simulink library "lib_Gimbal_Ctrl"  (R2017a)
settings: Solver=VariableStepAuto  StartTime=0.0  StopTime=10.0  RelTol=1e-3
undefined symbols (not defined in the file or in its folder): FT_HWI_CC_Data, Standard_Devices, UDP_Protocol
undefined symbols (not defined in the file): HIL_Data
libraries: simulink x19, sldrtlib x2
(part 1 of 2)
settings Model: Creator=m.hiepp  LastModifiedBy=m.hiepp
settings SFSimCC: SimUseLocalCustomCode=on
settings RTWCC: RTWUseLocalCustomCode=on

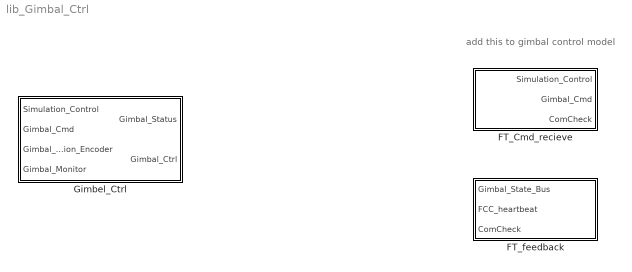
== system lib_Gimbal_Ctrl ==
  note: add this to gimbal control model
  FT_Cmd_recieve : Subsystem
  FT_feedback : Subsystem
  Gimbel_Ctrl : Subsystem  mask{Gimbal_Ctrl=HIL_Data.Gimbal_Ctrl, SampTime=HIL_Data.Gimbal_Ctrl.SampTime}
      mask prompts: SampTime "Sample Time"

== system lib_Gimbal_Ctrl/FT_Cmd_recieve ==
  note: serves also as hold when there is no new input!
  Construct_Busses : Subsystem
  Logical Operator : Logic  AllPortsSameDT=off  OutDataTypeStr=boolean
  NOT : Logic  Operator=NOT  IconShape=distinctive  AllPortsSameDT=off  OutDataTypeStr=boolean
  Receive_from_SimulationPC : sldrtlib/Packet Input  SampleTime=FT_HWI_CC_Data.SampTime  MaxMissedTicks=FT_HWI_CC_Data.MaxMissTicks  ShowMissedTicks=off  YieldWhenWaiting=on  DrvName=Standard_Devices/UDP_Protocol  DrvAddress=36880  DrvOptions=[3232235970 36864]  PacketSize=52  DataTypes={'boolean','boolean','double','double','uint16','double','double','double','double'}  ShowReady=on  ShowError=on  PacketID=1  ByteOrder=1  ShowTimestamp=off
      settings: AttributesFormatString=UDP Protocol [36880]  SourceProductName=Simulink Desktop Real-Time
  Simulation_Control : Outport  OutDataTypeStr=Bus: Simulation_Ctrl_Bus
  Gimbal_Cmd : Outport  Port=2  OutDataTypeStr=Bus: Gimbal_Cmd_Bus
  ComCheck : Outport  Port=3
  wires:
  Receive_from_SimulationPC/8 -> Construct_Busses/8(GimCmd_psi)  "Gimbal_Psi_Cmd_deg"
  Receive_from_SimulationPC/7 -> Construct_Busses/7(GimCmd_theta)  "Gimbal_Theta_Cmd_deg"
  Receive_from_SimulationPC/6 -> Construct_Busses/6(GimCmd_phi)  "Gimbal_Phi_Cmd_deg"
  Receive_from_SimulationPC/4 -> Construct_Busses/4(SimCtrl_gimbal_flg)  "stop_gimbal_flg"
  Receive_from_SimulationPC/3 -> Construct_Busses/3(SimCtrl_enable_gimbal_flg)  "enable_gimbal_ctrl_flg"
  Receive_from_SimulationPC/2 -> Construct_Busses/2(SimCtrl_reset)  "reset"
  Receive_from_SimulationPC/1 -> Construct_Busses/1(SimCtrl_run)  "run"
  Construct_Busses/2(Gimbal_Cmd) -> Gimbal_Cmd/1
  Construct_Busses/1(Simulation_Control) -> Simulation_Control/1
  Receive_from_SimulationPC/5 -> Construct_Busses/5(SimCtrl_heartbeat)  "Gimbal_Phi_Cmd_deg"
  NOT/1 -> Logical Operator/2
  Logical Operator/1 -> Construct_Busses/Enable
  Receive_from_SimulationPC/10 -> Logical Operator/1  "DataReady_flg"
  Receive_from_SimulationPC/11 -> NOT/1  "DataError_flg"
  Receive_from_SimulationPC/9 -> Construct_Busses/9(ComCheck_update)  "ComCheck"
  Construct_Busses/3(ComCheck) -> ComCheck/1

== system lib_Gimbal_Ctrl/FT_feedback ==
  note: only relevant signals are transfered
  Gimbal_State_Bus : Inport  OutDataTypeStr=Bus: Gimbal_State_Bus
  FCC_heartbeat : Inport  Port=2
  ComCheck : Inport  Port=3
  Bus Selector : BusSelector  OutputSignals=Gimbal_Status.Gimbal_operational_flg,Gimbal_Status.Gimbal_Ramp_flg,Gimbal_Status.Gimbal_Limit_flg,Gimbal_Status.Gimbal_StopSim_flg,Gimbal_Encoder_Signals.ATT_Gimbal.Gimbal_yaw_sns,Gimbal_Encoder_Signals.ATT_Gimbal.Gimbal_pitch_sns,Gimbal_Encoder_Signals.ATT_Gimbal.Gimbal_roll_sns
  Compare To Constant : simulink/Logic and Bit Operations/Compare To Constant  relop===  const=FT_HWI_CC_Data.ComFreq_mark  OutDataTypeStr=boolean
  Counter Limited : simulink/Sources/Counter Limited  uplimit=FT_HWI_CC_Data.ComFreq_mark  tsamp=FT_HWI_CC_Data.SampTime
  send_FB : Subsystem
  wires:
  Gimbal_State_Bus/1 -> Bus Selector/1
  Counter Limited/1 -> Compare To Constant/1
  Bus Selector/1 -> send_FB/1(Gimbal_operational_flg)  "<Gimbal_operational_flg>"
  Bus Selector/2 -> send_FB/2(Gimbal_Ramp_flg)  "<Gimbal_Ramp_flg>"
  Bus Selector/3 -> send_FB/3(Gimbal_Limit_flg)  "<Gimbal_Limit_flg>"
  Bus Selector/4 -> send_FB/4(Gimbal_StopSim_flg)  "<Gimbal_StopSim_flg>"
  Bus Selector/5 -> send_FB/5(Gimbal_yaw_sns)  "<Gimbal_yaw_sns>"
  Bus Selector/6 -> send_FB/6(Gimbal_pitch_sns)  "<Gimbal_pitch_sns>"
  Bus Selector/7 -> send_FB/7(Gimbal_roll_sns)  "<Gimbal_roll_sns>"
  Compare To Constant/1 -> send_FB/Enable
  FCC_heartbeat/1 -> send_FB/8(FCC_heartbeat)
  ComCheck/1 -> send_FB/9(ComCheck)

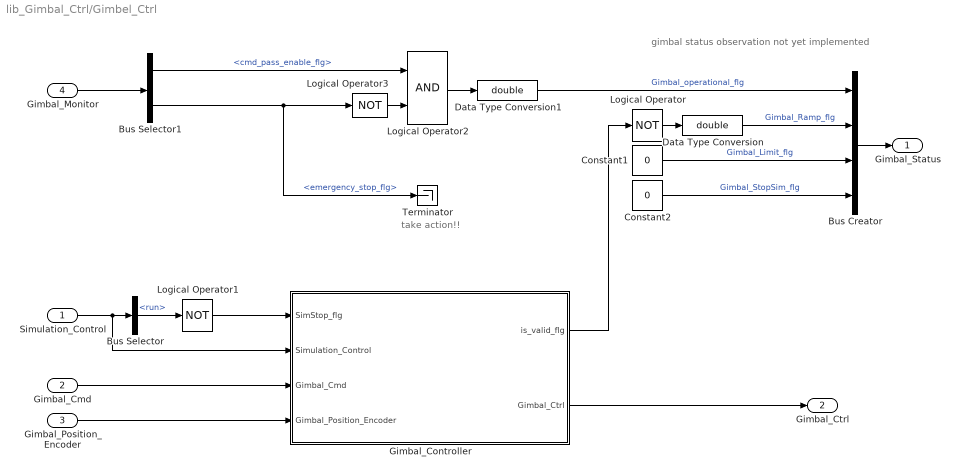
== system lib_Gimbal_Ctrl/Gimbel_Ctrl ==
  note: take action!!
  note: gimbal status observation not yet implemented
  Simulation_Control : Inport  OutDataTypeStr=Bus: Simulation_Ctrl_Bus
  Gimbal_Cmd : Inport  Port=2  OutDataTypeStr=Bus: Gimbal_Cmd_Bus
  Gimbal_Position_Encoder : Inport  Port=3  OutDataTypeStr=Bus: Gimbal_Encoder_Bus
  Gimbal_Monitor : Inport  Port=4  OutDataTypeStr=Bus: Gimbal_Monitor_Bus
  Bus Creator : BusCreator  Inputs=4
  Bus Selector : BusSelector  OutputSignals=run
  Bus Selector1 : BusSelector  OutputSignals=cmd_pass_enable_flg,emergency_stop_flg
  Constant1 : Constant  Value=0
  Constant2 : Constant  Value=0
  Data Type Conversion : DataTypeConversion  OutDataTypeStr=double
  Data Type Conversion1 : DataTypeConversion  OutDataTypeStr=double
  Gimbal_Controller : Subsystem
  Logical Operator : Logic  Operator=NOT  AllPortsSameDT=off  OutDataTypeStr=boolean
  Logical Operator1 : Logic  Operator=NOT  AllPortsSameDT=off  OutDataTypeStr=boolean
  Logical Operator2 : Logic  AllPortsSameDT=off  OutDataTypeStr=boolean
  Logical Operator3 : Logic  Operator=NOT  AllPortsSameDT=off  OutDataTypeStr=boolean
  Terminator : Terminator
  Gimbal_Status : Outport  OutDataTypeStr=Bus: Gimbal_Status_Bus
  Gimbal_Ctrl : Outport  Port=2  OutDataTypeStr=Bus: Gimbal_Ctrl_Bus
  wires:
  Bus Creator/1 -> Gimbal_Status/1
  Logical Operator/1 -> Data Type Conversion/1
  Gimbal_Controller/2(Gimbal_Ctrl) -> Gimbal_Ctrl/1
  Gimbal_Controller/1(is_valid_flg) -> Logical Operator/1
  Simulation_Control/1 -> Gimbal_Controller/2(Simulation_Control), Bus Selector/1
  Gimbal_Position_Encoder/1 -> Gimbal_Controller/4(Gimbal_Position_Encoder)
  Gimbal_Cmd/1 -> Gimbal_Controller/3(Gimbal_Cmd)
  Bus Selector/1 -> Logical Operator1/1  "<run>"
  Logical Operator1/1 -> Gimbal_Controller/1(SimStop_flg)
  Data Type Conversion1/1 -> Bus Creator/1  "Gimbal_operational_flg"
  Constant1/1 -> Bus Creator/3  "Gimbal_Limit_flg"
  Constant2/1 -> Bus Creator/4  "Gimbal_StopSim_flg"
  Data Type Conversion/1 -> Bus Creator/2  "Gimbal_Ramp_flg"
  Gimbal_Monitor/1 -> Bus Selector1/1
  Bus Selector1/1 -> Logical Operator2/1  "<cmd_pass_enable_flg>"
  Bus Selector1/2 -> Terminator/1, Logical Operator3/1  "<emergency_stop_flg>"
  Logical Operator2/1 -> Data Type Conversion1/1
  Logical Operator3/1 -> Logical Operator2/2

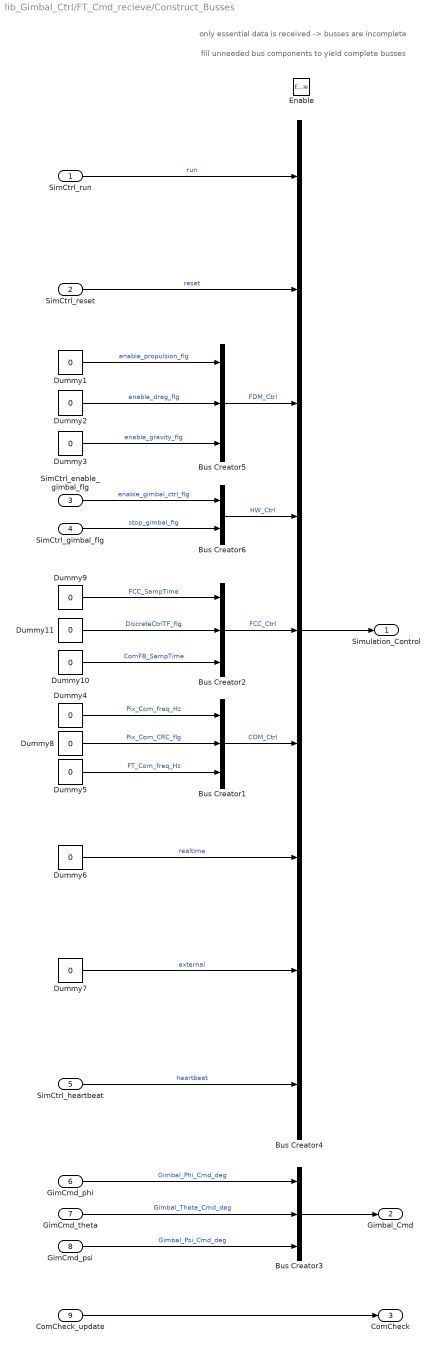
== system lib_Gimbal_Ctrl/FT_Cmd_recieve/Construct_Busses ==
  note: only essential data is received -> busses are incomplete
  note: fill unneeded bus components to yield complete busses
  SimCtrl_run : Inport
  SimCtrl_reset : Inport  Port=2
  SimCtrl_enable_gimbal_flg : Inport  Port=3
  SimCtrl_gimbal_flg : Inport  Port=4
  SimCtrl_heartbeat : Inport  Port=5
  GimCmd_phi : Inport  Port=6
  GimCmd_theta : Inport  Port=7
  GimCmd_psi : Inport  Port=8
  ComCheck_update : Inport  Port=9
  Enable : EnablePort
  Bus Creator1 : BusCreator  Inputs=3  OutDataTypeStr=Bus: COM_Ctrl_Bus
  Bus Creator2 : BusCreator  Inputs=3  OutDataTypeStr=Bus: FCC_Ctrl_Bus
  Bus Creator3 : BusCreator  Inputs=3  OutDataTypeStr=Bus: Gimbal_Cmd_Bus
  Bus Creator4 : BusCreator  Inputs=9  OutDataTypeStr=Bus: Simulation_Ctrl_Bus
  Bus Creator5 : BusCreator  Inputs=3  OutDataTypeStr=Bus: FDM_Ctrl_Bus
  Bus Creator6 : BusCreator  Inputs=2  OutDataTypeStr=Bus: HW_Ctrl_Bus
  Dummy{1..3,6..8,11} (7 alike) : Constant  Value=0  OutDataTypeStr=boolean
  Dummy{4..5,9..10} (4 alike) : Constant  Value=0  OutDataTypeStr=double
  Simulation_Control : Outport  OutDataTypeStr=Bus: Simulation_Ctrl_Bus
  Gimbal_Cmd : Outport  Port=2  OutDataTypeStr=Bus: Gimbal_Cmd_Bus
  ComCheck : Outport  Port=3
  wires:
  GimCmd_phi/1 -> Bus Creator3/1  "Gimbal_Phi_Cmd_deg"
  GimCmd_psi/1 -> Bus Creator3/3  "Gimbal_Psi_Cmd_deg"
  GimCmd_theta/1 -> Bus Creator3/2  "Gimbal_Theta_Cmd_deg"
  Bus Creator3/1 -> Gimbal_Cmd/1
  SimCtrl_gimbal_flg/1 -> Bus Creator6/2  "stop_gimbal_flg"
  SimCtrl_enable_gimbal_flg/1 -> Bus Creator6/1  "enable_gimbal_ctrl_flg"
  Bus Creator6/1 -> Bus Creator4/4  "HW_Ctrl"
  Bus Creator5/1 -> Bus Creator4/3  "FDM_Ctrl"
  Dummy3/1 -> Bus Creator5/3  "enable_gravity_flg"
  Dummy2/1 -> Bus Creator5/2  "enable_drag_flg"
  Dummy1/1 -> Bus Creator5/1  "enable_propulsion_flg"
  SimCtrl_run/1 -> Bus Creator4/1  "run"
  Bus Creator4/1 -> Simulation_Control/1
  SimCtrl_heartbeat/1 -> Bus Creator4/9  "heartbeat"
  Dummy7/1 -> Bus Creator4/8  "external"
  Dummy6/1 -> Bus Creator4/7  "realtime"
  Bus Creator1/1 -> Bus Creator4/6  "COM_Ctrl"
  SimCtrl_reset/1 -> Bus Creator4/2  "reset"
  Dummy4/1 -> Bus Creator1/1  "Pix_Com_freq_Hz"
  Dummy5/1 -> Bus Creator1/3  "FT_Com_freq_Hz"
  Dummy8/1 -> Bus Creator1/2  "Pix_Com_CRC_flg"
  Bus Creator2/1 -> Bus Creator4/5  "FCC_Ctrl"
  Dummy11/1 -> Bus Creator2/2  "DiscreteCtrlTF_flg"
  Dummy9/1 -> Bus Creator2/1  "FCC_SampTime"
  Dummy10/1 -> Bus Creator2/3  "ComFB_SampTime"
  ComCheck_update/1 -> ComCheck/1

== system lib_Gimbal_Ctrl/FT_feedback/send_FB ==
  Gimbal_operational_flg : Inport
  Gimbal_Ramp_flg : Inport  Port=2
  Gimbal_Limit_flg : Inport  Port=3
  Gimbal_StopSim_flg : Inport  Port=4
  Gimbal_yaw_sns : Inport  Port=5
  Gimbal_pitch_sns : Inport  Port=6
  Gimbal_roll_sns : Inport  Port=7
  FCC_heartbeat : Inport  Port=8
  ComCheck : Inport  Port=9
  Enable : EnablePort
  Feddback_to_SimPC : sldrtlib/Packet Output  SampleTime=FT_HWI_CC_Data.SampTime  MaxMissedTicks=FT_HWI_CC_Data.MaxMissedTicks  ShowMissedTicks=off  YieldWhenWaiting=on  DrvName=Standard_Devices/UDP_Protocol  DrvAddress=36864  DrvOptions=[0 36880 49 57 50 46 49 54 56 46 49 46 49 53 54 0 0 0 0 0 0 0 0 0 0 0 0 0 0 0 0 0 0 0 0 0 0 0 0 0 0 0 0 0 0 0 0 0 0 0 0 0 0 0 0 0 0 0 0 0 0 0 0 0 0 0 0 0 0 0 0 0 0 0 0 0 0 0 0 0 0 0 0 0 0 0 0 0 0 0 0 0 0 0 0 0 0 0 0 0 0 0 0 0 0 0 0 0 0 0 0 0 0 0 0 0 0 0 0 0 0 0 0 0 0 0 0 0 0 0 0 0 0 0 0 0 0 0 0 0 0 0 0 0 0 0 0 0 0 0 0 0 0 0 0 0 0 0 0 0 0 0 0 0 0 0 0 0 0 0 0 0 0 0 0 0 0 0 0 0 0 0 0 0 0 0 0 0 0 0 0 0 0 0 0 0 0 0 0 0 0 0 0 0 0 0 0 0 0 0 0 0 0 0 0 0 0 0 0 0 0 0 0 0 0 0 0 0 0 0 0 0 0 0 0 0 0 0 0 0 0 0 0 0 0 0 0 0 0 0 0 0 0 0 0 0]  PacketSize=66  DataTypes={'double','double','double','double','double','double','double','uint16','double'}  ShowReady=off  ShowError=off  PacketID=1  ByteOrder=1  InitialValue=[]  FinalValue=[]
      settings: AttributesFormatString=UDP Protocol [36864]  SourceProductName=Simulink Desktop Real-Time
  wires:
  Gimbal_operational_flg/1 -> Feddback_to_SimPC/1
  Gimbal_yaw_sns/1 -> Feddback_to_SimPC/5
  Gimbal_StopSim_flg/1 -> Feddback_to_SimPC/4
  Gimbal_Ramp_flg/1 -> Feddback_to_SimPC/2
  Gimbal_Limit_flg/1 -> Feddback_to_SimPC/3
  Gimbal_pitch_sns/1 -> Feddback_to_SimPC/6
  Gimbal_roll_sns/1 -> Feddback_to_SimPC/7
  FCC_heartbeat/1 -> Feddback_to_SimPC/8
  ComCheck/1 -> Feddback_to_SimPC/9

== system lib_Gimbal_Ctrl/Gimbel_Ctrl/Gimbal_Controller ==
  note: this is a copy of the controller run on the gimbal control PC
  note: keep it up to date!!!
  note: adapt constant names to struct names!!
  SimStop_flg : Inport
  Simulation_Control : Inport  Port=2  OutDataTypeStr=Bus: Simulation_Ctrl_Bus
  Gimbal_Cmd : Inport  Port=3  OutDataTypeStr=Bus: Gimbal_Cmd_Bus
  Gimbal_Position_Encoder : Inport  Port=4  OutDataTypeStr=Bus: Gimbal_Encoder_Bus
  Bus Creator : BusCreator  Inputs=5  OutDataTypeStr=Bus: Gimbal_Ctrl_Bus
  Bus Selector : BusSelector  OutputSignals=Gimbal_Phi_Cmd_deg,Gimbal_Theta_Cmd_deg,Gimbal_Psi_Cmd_deg
  Bus Selector1 : BusSelector  OutputSignals=ATT_Gimbal.Gimbal_yaw_sns,ATT_Gimbal.Gimbal_pitch_sns,ATT_Gimbal.Gimbal_roll_sns
  Bus Selector2 : BusSelector  OutputSignals=HW_Ctrl.enable_gimbal_ctrl_flg,HW_Ctrl.stop_gimbal_flg
  Controller : Subsystem
  Gain : Gain
  Gain1 : Gain
  is_valid_flg : Outport
  Gimbal_Ctrl : Outport  Port=2  OutDataTypeStr=Bus: Gimbal_Ctrl_Bus
  wires:
  Bus Creator/1 -> Gimbal_Ctrl/1
  Gimbal_Cmd/1 -> Bus Selector/1
  Gimbal_Position_Encoder/1 -> Bus Selector1/1
  SimStop_flg/1 -> Controller/4(Stop_flg)
  Controller/4(is_valid_flg) -> is_valid_flg/1
  Bus Selector1/1 -> Controller/1(Yaw_sns)  "<Gimbal_yaw_sns>"
  Bus Selector1/2 -> Controller/2(pitch_sns)  "<Gimbal_pitch_sns>"
  Bus Selector1/3 -> Controller/3(roll_sns)  "<Gimbal_roll_sns>"
  Bus Selector/1 -> Controller/5(Yaw_Cmd_deg)  "<Gimbal_Phi_Cmd_deg>"
  Bus Selector/2 -> Controller/6(Pitch_Cmd_deg)  "<Gimbal_Theta_Cmd_deg>"
  Bus Selector/3 -> Controller/7(Roll_Cmd_deg)  "<Gimbal_Psi_Cmd_deg>"
  Controller/1(Roll2motor) -> Bus Creator/3  "Gimbal_Phi2Motor"
  Controller/2(Pitch2motor) -> Bus Creator/4  "Gimbal_Theta2Motor"
  Controller/3(Yaw2motor) -> Bus Creator/5  "Gimbal_Psi2Motor"
  Simulation_Control/1 -> Bus Selector2/1
  Bus Selector2/1 -> Gain/1  "<enable_gimbal_ctrl_flg>"
  Bus Selector2/2 -> Gain1/1  "<stop_gimbal_flg>"
  Gain/1 -> Bus Creator/1  "enable_gimbal_ctrl_flg"
  Gain1/1 -> Bus Creator/2  "stop_gimbal_flg"

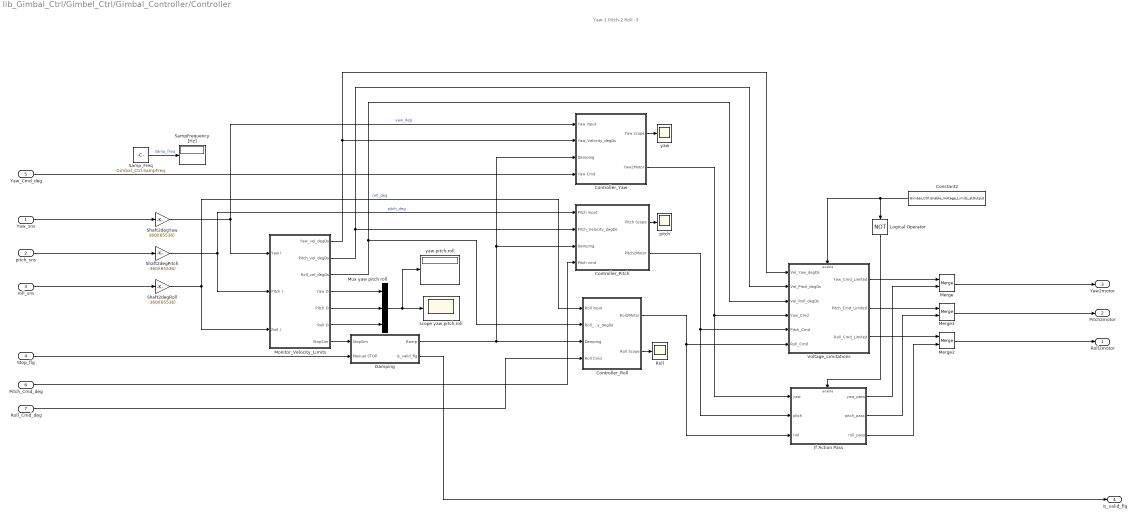
== system lib_Gimbal_Ctrl/Gimbel_Ctrl/Gimbal_Controller/Controller ==
  note: Yaw-1
      | Pitch-2
      | Roll -3
  Yaw_sns : Inport
  pitch_sns : Inport  Port=2
  roll_sns : Inport  Port=3
  Stop_flg : Inport  Port=4
  Yaw_Cmd_deg : Inport  Port=5
  Pitch_Cmd_deg : Inport  Port=6
  Roll_Cmd_deg : Inport  Port=7
  Constant2 : Constant  Value=Gimbal_Ctrl.Enable_Voltage_Limits_atOutput
  Controller_Pitch : Subsystem
      mask Display:
      | disp('Pitch - 2')
      | set_param(gcb,'BackgroundColor','cyan')
      | port_label('input',1,'Pitch input')
      | port_label('input',3,'Damping')
      | port_label('input',2,'Pitch Vel')
      | port_label('input',4,'Pitch Cmd')
      | port_label('output',1,'Pitch scope')
      | port_label('output',2,'Pitch2Motor')
  Controller_Roll : Subsystem
      mask Display:
      | disp('Roll - 3')
      | set_param(gcb,'BackgroundColor','Orange')
      | port_label('input',1,'Roll input')
      | port_label('input',3,'Damping')
      | port_label('input',2,'Roll Vel')
      | port_label('input',4,'Roll Cmd')
      | port_label('output',2,'Roll scope')
      | port_label('output',1,'Roll2Motor')
  Controller_Yaw : Subsystem
      mask Display:
      | disp('Yaw - 1')
      | set_param(gcb,'BackgroundColor','Yellow')
      | port_label('input',1,'Yaw input')
      | port_label('input',2,'Yaw Vel')
      | port_label('input',3,'Damping')
      | port_label('input',4,'Yaw Cmd')
      | port_label('output',1,'Yaw scope')
      | port_label('output',2,'Yaw2Motor')
  Damping : Subsystem
  If Action Pass : Subsystem  TreatAsAtomicUnit=on
  Logical Operator : Logic  Operator=NOT  AllPortsSameDT=off  OutDataTypeStr=boolean
  Merge : Merge
  Merge1 : Merge
  Merge2 : Merge
  Monitor_Velocity_Limits : Subsystem
  Mux yaw pitch roll : Mux  Inputs=3
  Roll : Scope
  SampFrequency [Hz] : Display
      settings: Tag=SampTime
  Samp_Freq : Constant  Value=Gimbal_Ctrl.SampFreq
  Shaft2degPitch : Gain  Gain=-360/(65536)
  Shaft2degRoll : Gain  Gain=-360/(65536)
  Shaft2degYaw : Gain  Gain=360/(65536)
  Voltage_Limitations : Subsystem
  pitch : Scope
  scope yaw,pitch,roll : Scope
  yaw : Scope
  yaw,pitch,roll : Display
      settings: Tag=yaw pitch roll
  Roll2motor : Outport
  Pitch2motor : Outport  Port=2
  Yaw2motor : Outport  Port=3
  is_valid_flg : Outport  Port=4
  wires:
  Merge2/1 -> Roll2motor/1
  Voltage_Limitations/3(Roll_Cmd_Limited) -> Merge2/1
  Damping/2(is_valid_flg) -> is_valid_flg/1
  Yaw_Cmd_deg/1 -> Controller_Yaw/4(Yaw Cmd)
  Shaft2degRoll/1 -> Controller_Roll/1(Roll input), Monitor_Velocity_Limits/3(Roll I)  "roll_deg"
  Controller_Yaw/1("Yaw scope ") -> yaw/1
  Monitor_Velocity_Limits/4(Yaw O) -> Mux yaw pitch roll/1
  Shaft2degYaw/1 -> Controller_Yaw/1(Yaw input), Monitor_Velocity_Limits/1(Yaw I)  "yaw_deg"
  Controller_Yaw/2(Yaw2Motor) -> Voltage_Limitations/4(Yaw_Cmd), If Action Pass/1(yaw)
  Monitor_Velocity_Limits/2(Pitch_vel_degDs) -> Voltage_Limitations/2(Vel_Pitch_degDs), Controller_Pitch/2(Pitch_Velocity_degDs)
  Damping/1(Ramp) -> Controller_Roll/3(Damping), Controller_Pitch/3(Damping), Controller_Yaw/3(Damping)
  Monitor_Velocity_Limits/3(Roll_vel_degDs) -> Voltage_Limitations/3(Vel_Roll_degDs), Controller_Roll/2(Roll_Velocity_degDs)
  Pitch_Cmd_deg/1 -> Controller_Pitch/4(Pitch cmd)
  Voltage_Limitations/2(Pitch_Cmd_Limited) -> Merge1/1
  Mux yaw pitch roll/1 -> yaw,pitch,roll/1, scope yaw,pitch,roll/1
  pitch_sns/1 -> Shaft2degPitch/1
  Controller_Roll/2(Roll Scope) -> Roll/1
  Controller_Pitch/1(Pitch Scope) -> pitch/1
  Constant2/1 -> Voltage_Limitations/Enable, Logical Operator/1
  Monitor_Velocity_Limits/5(Pitch O) -> Mux yaw pitch roll/2
  Voltage_Limitations/1(Yaw_Cmd_Limited) -> Merge/1
  Monitor_Velocity_Limits/7(StopSim) -> Damping/1(StopSim)
  Controller_Roll/1(Roll2Motor) -> Voltage_Limitations/6(Roll_Cmd), If Action Pass/3(roll)
  Shaft2degPitch/1 -> Monitor_Velocity_Limits/2(Pitch I), Controller_Pitch/1("Pitch input ")  "pitch_deg"
  Monitor_Velocity_Limits/1(Yaw_vel_degDs) -> Controller_Yaw/2(Yaw_Velocity_degDs), Voltage_Limitations/1(Vel_Yaw_degDs)
  Controller_Pitch/2(Pitch2Motor) -> Voltage_Limitations/5(Pitch_Cmd), If Action Pass/2(pitch)
  Merge1/1 -> Pitch2motor/1
  Merge/1 -> Yaw2motor/1
  Monitor_Velocity_Limits/6(Roll O) -> Mux yaw pitch roll/3
  Stop_flg/1 -> Damping/2(Manual STOP)
  Logical Operator/1 -> If Action Pass/Enable
  If Action Pass/3(roll_pass) -> Merge2/2
  If Action Pass/1(yaw_pass) -> Merge/2
  Roll_Cmd_deg/1 -> Controller_Roll/4(Roll Cmd)
  If Action Pass/2(pitch_pass) -> Merge1/2
  Yaw_sns/1 -> Shaft2degYaw/1
  Samp_Freq/1 -> SampFrequency [Hz]/1  "Samp_freq"
  roll_sns/1 -> Shaft2degRoll/1

== system lib_Gimbal_Ctrl/Gimbel_Ctrl/Gimbal_Controller/Controller/Controller_Pitch ==
  "Pitch input " : Inport
  Pitch_Velocity_degDs : Inport  Port=2
  Damping : Inport  Port=3
  Pitch cmd : Inport  Port=4
  Limits : Subsystem
  Mux pitch : Mux  Inputs=3
  PID Controller Pitch : simulink/Continuous/PID Controller  Commented=on  Controller=PID  Form=Parallel  TimeDomain=Continuous-time  SampleTime=-1  IntegratorMethod=Forward Euler  FilterMethod=Forward Euler  ControllerParametersSource=internal  P=20  I=0  D=0.4  UseFilter=on  N=100  InitialConditionSource=internal  InitialConditionForIntegrator=0  InitialConditionForFilter=0  DifferentiatorICPrevScaledInput=0  ExternalReset=none  TrackingMode=off  Kt=1  LimitOutput=off  UpperSaturationLimit=inf  LowerSaturationLimit=-inf  LinearizeAsGain=on  AntiWindupMode=none  Kb=1  POutMin=[]  POutMax=[]  IOutMin=[]  IOutMax=[]  DOutMin=[]  DOutMax=[]  NOutMin=[]  NOutMax=[]  SumOutMin=[]  SumOutMax=[]  SaturationOutMin=[]  SaturationOutMax=[]  PParamMin=[]  PParamMax=[]  IParamMin=[]  IParamMax=[]  DParamMin=[]  DParamMax=[]  NParamMin=[]  NParamMax=[]  KbParamMin=[]  KbParamMax=[]  KtParamMin=[]  KtParamMax=[]  KbOutMin=[]  KbOutMax=[]  KtOutMin=[]  KtOutMax=[]  IntegratorOutMin=[]  IntegratorOutMax=[]  FilterOutMin=[]  FilterOutMax=[]  SumI1OutMin=[]  SumI1OutMax=[]  SumI2OutMin=[]  SumI2OutMax=[]  SumI3OutMin=[]  SumI3OutMax=[]  SumDOutMin=[]  SumDOutMax=[]  DifferentiatorOutMin=[]  DifferentiatorOutMax=[]  IntegratorContinuousStateAttributes=''  IntegratorStateMustResolveToSignalObject=off  IntegratorRTWStateStorageClass=Auto  FilterContinuousStateAttributes=''  FilterStateMustResolveToSignalObject=off  FilterRTWStateStorageClass=Auto
  PID_Controller_Dynamic_Limits : Subsystem
  Product : Product
  Sum2 : Sum  Inputs=+-|
  Pitch Scope : Outport
  Pitch2Motor : Outport  Port=2
  wires:
  PID_Controller_Dynamic_Limits/1(Controller_Output) -> Pitch2Motor/1  "pitch2motor"
  Sum2/1 -> PID_Controller_Dynamic_Limits/1(Error_Signal_Input), Mux pitch/3  "pitch_err"
  Product/1 -> Mux pitch/2, Sum2/1  "pitch_cmd"
  Mux pitch/1 -> Pitch Scope/1
  Pitch cmd/1 -> Product/2
  "Pitch input "/1 -> Mux pitch/1, Sum2/2
  Damping/1 -> Product/1
  Limits/3(lower_limit) -> PID_Controller_Dynamic_Limits/4(lower_limit_output)
  Limits/2(upper_limit) -> PID_Controller_Dynamic_Limits/3(upper_limit_output)
  Limits/1(limit_flg) -> PID_Controller_Dynamic_Limits/2(limit_output_flg)
  Pitch_Velocity_degDs/1 -> Limits/1(velocity)

== system lib_Gimbal_Ctrl/Gimbel_Ctrl/Gimbal_Controller/Controller/Controller_Roll ==
  Roll input : Inport
  Roll_Velocity_degDs : Inport  Port=2
  Damping : Inport  Port=3
  Roll Cmd : Inport  Port=4
  Limits : Subsystem
  PID Controller Roll : simulink/Continuous/PID Controller  Commented=on  Controller=PID  Form=Parallel  TimeDomain=Continuous-time  SampleTime=-1  IntegratorMethod=Forward Euler  FilterMethod=Forward Euler  ControllerParametersSource=internal  P=8  I=0.2  D=0.35  UseFilter=on  N=100  InitialConditionSource=internal  InitialConditionForIntegrator=0  InitialConditionForFilter=0  DifferentiatorICPrevScaledInput=0  ExternalReset=none  TrackingMode=off  Kt=1  LimitOutput=off  UpperSaturationLimit=inf  LowerSaturationLimit=-inf  LinearizeAsGain=on  AntiWindupMode=none  Kb=1  POutMin=[]  POutMax=[]  IOutMin=[]  IOutMax=[]  DOutMin=[]  DOutMax=[]  NOutMin=[]  NOutMax=[]  SumOutMin=[]  SumOutMax=[]  SaturationOutMin=[]  SaturationOutMax=[]  PParamMin=[]  PParamMax=[]  IParamMin=[]  IParamMax=[]  DParamMin=[]  DParamMax=[]  NParamMin=[]  NParamMax=[]  KbParamMin=[]  KbParamMax=[]  KtParamMin=[]  KtParamMax=[]  KbOutMin=[]  KbOutMax=[]  KtOutMin=[]  KtOutMax=[]  IntegratorOutMin=[]  IntegratorOutMax=[]  FilterOutMin=[]  FilterOutMax=[]  SumI1OutMin=[]  SumI1OutMax=[]  SumI2OutMin=[]  SumI2OutMax=[]  SumI3OutMin=[]  SumI3OutMax=[]  SumDOutMin=[]  SumDOutMax=[]  DifferentiatorOutMin=[]  DifferentiatorOutMax=[]  IntegratorContinuousStateAttributes=''  IntegratorStateMustResolveToSignalObject=off  IntegratorRTWStateStorageClass=Auto  FilterContinuousStateAttributes=''  FilterStateMustResolveToSignalObject=off  FilterRTWStateStorageClass=Auto
  PID_Controller_Dynamic_Limits : Subsystem
  Product1 : Product
  Roll yaw : Mux  Inputs=3
  Sum1 : Sum  Inputs=+-|
  XY Graph Roll : simulink/Sinks/XY Graph  Commented=on  xmin=-40  xmax=40  ymin=-40  ymax=40  st=-1
  Roll2Motor : Outport
  Roll Scope : Outport  Port=2
  wires:
  Roll input/1 -> XY Graph Roll/1, Roll yaw/2, Sum1/2
  PID_Controller_Dynamic_Limits/1(Controller_Output) -> Roll2Motor/1  "roll2motor"
  Sum1/1 -> PID_Controller_Dynamic_Limits/1(Error_Signal_Input), Roll yaw/3  "Roll_err"
  Roll yaw/1 -> Roll Scope/1
  Product1/1 -> Roll yaw/1, XY Graph Roll/2, Sum1/1
  Damping/1 -> Product1/1
  Roll Cmd/1 -> Product1/2
  Limits/3(lower_limit) -> PID_Controller_Dynamic_Limits/4(lower_limit_output)
  Limits/2(upper_limit) -> PID_Controller_Dynamic_Limits/3(upper_limit_output)
  Limits/1(limit_flg) -> PID_Controller_Dynamic_Limits/2(limit_output_flg)
  Roll_Velocity_degDs/1 -> Limits/1(velocity)

== system lib_Gimbal_Ctrl/Gimbel_Ctrl/Gimbal_Controller/Controller/Controller_Yaw ==
  Yaw input : Inport
  Yaw_Velocity_degDs : Inport  Port=2
  Damping : Inport  Port=3
  Yaw Cmd : Inport  Port=4
  Limit_Controllers : Subsystem
  Limits : Subsystem
  Mux yaw : Mux  Inputs=3
  PID Controller Yaw : simulink/Continuous/PID Controller  Commented=on  Controller=PID  Form=Parallel  TimeDomain=Continuous-time  SampleTime=-1  IntegratorMethod=Forward Euler  FilterMethod=Forward Euler  ControllerParametersSource=internal  P=3  I=0.1  D=0.4  UseFilter=on  N=100  InitialConditionSource=internal  InitialConditionForIntegrator=0  InitialConditionForFilter=0  DifferentiatorICPrevScaledInput=0  ExternalReset=none  TrackingMode=off  Kt=1  LimitOutput=off  UpperSaturationLimit=inf  LowerSaturationLimit=-inf  LinearizeAsGain=on  AntiWindupMode=none  Kb=1  POutMin=[]  POutMax=[]  IOutMin=[]  IOutMax=[]  DOutMin=[]  DOutMax=[]  NOutMin=[]  NOutMax=[]  SumOutMin=[]  SumOutMax=[]  SaturationOutMin=[]  SaturationOutMax=[]  PParamMin=[]  PParamMax=[]  IParamMin=[]  IParamMax=[]  DParamMin=[]  DParamMax=[]  NParamMin=[]  NParamMax=[]  KbParamMin=[]  KbParamMax=[]  KtParamMin=[]  KtParamMax=[]  KbOutMin=[]  KbOutMax=[]  KtOutMin=[]  KtOutMax=[]  IntegratorOutMin=[]  IntegratorOutMax=[]  FilterOutMin=[]  FilterOutMax=[]  SumI1OutMin=[]  SumI1OutMax=[]  SumI2OutMin=[]  SumI2OutMax=[]  SumI3OutMin=[]  SumI3OutMax=[]  SumDOutMin=[]  SumDOutMax=[]  DifferentiatorOutMin=[]  DifferentiatorOutMax=[]  IntegratorContinuousStateAttributes=''  IntegratorStateMustResolveToSignalObject=off  IntegratorRTWStateStorageClass=Auto  FilterContinuousStateAttributes=''  FilterStateMustResolveToSignalObject=off  FilterRTWStateStorageClass=Auto
  PID_Controller_Dynamic_Limits : Subsystem
  Product : Product
  Sum : Sum  Inputs=+-|
  XY Graph yaw : simulink/Sinks/XY Graph  Commented=on  xmin=-40  xmax=40  ymin=-40  ymax=40  st=-1
  "Yaw scope " : Outport
  Yaw2Motor : Outport  Port=2
  wires:
  Sum/1 -> PID_Controller_Dynamic_Limits/1(Error_Signal_Input), Mux yaw/3  "Yaw_err"
  Mux yaw/1 -> "Yaw scope "/1
  Yaw input/1 -> Mux yaw/2, XY Graph yaw/1, Sum/2
  Damping/1 -> Product/1
  Product/1 -> XY Graph yaw/2, Mux yaw/1, Sum/1
  Yaw Cmd/1 -> Product/2
  Yaw_Velocity_degDs/1 -> Limit_Controllers/2(Velocity), Limits/1(velocity)
  Limits/1(limit_flg) -> PID_Controller_Dynamic_Limits/2(limit_output_flg)
  Limits/2(upper_limit) -> PID_Controller_Dynamic_Limits/3(upper_limit_output)
  Limits/3(lower_limit) -> PID_Controller_Dynamic_Limits/4(lower_limit_output)
  PID_Controller_Dynamic_Limits/1(Controller_Output) -> Limit_Controllers/1(Controller_Cmd)
  Limit_Controllers/1(Output) -> Yaw2Motor/1

== system lib_Gimbal_Ctrl/Gimbel_Ctrl/Gimbal_Controller/Controller/Damping ==
  StopSim : Inport
  Manual STOP : Inport  Port=2
  Abs : Abs
  Compare To Constant : simulink/Logic and Bit Operations/Compare To Constant  relop=<  const=0.01  OutDataTypeStr=boolean
  Constant2 : Constant
  Data Type Conversion : DataTypeConversion  OutDataTypeStr=double
  Logical Operator : Logic  Operator=OR  AllPortsSameDT=off  OutDataTypeStr=boolean
  Logical Operator1 : Logic  Operator=NOT  AllPortsSameDT=off  OutDataTypeStr=boolean
  Subtract : Sum  Inputs=+-
  Transfer Fcn1 : TransferFcn  Numerator=[0.25]  Denominator=[1 1 0.25]
  Ramp : Outport
  is_valid_flg : Outport  Port=2
  wires:
  Transfer Fcn1/1 -> Ramp/1, Subtract/1
  Compare To Constant/1 -> is_valid_flg/1
  Subtract/1 -> Abs/1
  Constant2/1 -> Subtract/2
  Abs/1 -> Compare To Constant/1
  Data Type Conversion/1 -> Transfer Fcn1/1
  Logical Operator1/1 -> Data Type Conversion/1
  Logical Operator/1 -> Logical Operator1/1
  StopSim/1 -> Logical Operator/1
  Manual STOP/1 -> Logical Operator/2

== system lib_Gimbal_Ctrl/Gimbel_Ctrl/Gimbal_Controller/Controller/If Action Pass ==
  yaw : Inport
  pitch : Inport  Port=2
  roll : Inport  Port=3
  Enable : EnablePort
  yaw_pass : Outport
  pitch_pass : Outport  Port=2
  roll_pass : Outport  Port=3
  wires:
  yaw/1 -> yaw_pass/1
  pitch/1 -> pitch_pass/1
  roll/1 -> roll_pass/1

== system lib_Gimbal_Ctrl/Gimbel_Ctrl/Gimbal_Controller/Controller/Monitor_Velocity_Limits ==
  Yaw I : Inport
  Pitch I : Inport  Port=2
  Roll I : Inport  Port=3
  Logical Operator : Logic  Operator=OR  Inputs=3  AllPortsSameDT=off  OutDataTypeStr=boolean
  Pitch_rate_limit : Subsystem
  Roll_Rate_limit : Subsystem
  Yaw_rate_limit : Subsystem
  Yaw_vel_degDs : Outport
  Pitch_vel_degDs : Outport  Port=2
  Roll_vel_degDs : Outport  Port=3
  Yaw O : Outport  Port=4
  Pitch O : Outport  Port=5
  Roll O : Outport  Port=6
  StopSim : Outport  Port=7
  wires:
  Pitch_rate_limit/2(StopSim) -> Logical Operator/1
  Yaw_rate_limit/3(Continue) -> Yaw O/1
  Pitch_rate_limit/3(Continue) -> Pitch O/1
  Roll_Rate_limit/2(StopSim) -> Logical Operator/2
  Yaw_rate_limit/2(StopSim) -> Logical Operator/3
  Roll_Rate_limit/3(Continue) -> Roll O/1
  Yaw I/1 -> Yaw_rate_limit/1("Input ")
  Pitch I/1 -> Pitch_rate_limit/1("Input ")
  Roll I/1 -> Roll_Rate_limit/1("Input ")
  Logical Operator/1 -> StopSim/1
  Yaw_rate_limit/1(Yaw_vel_degDs) -> Yaw_vel_degDs/1
  Pitch_rate_limit/1(Pitch_vel_degDs) -> Pitch_vel_degDs/1
  Roll_Rate_limit/1(Roll_vel_degDs) -> Roll_vel_degDs/1

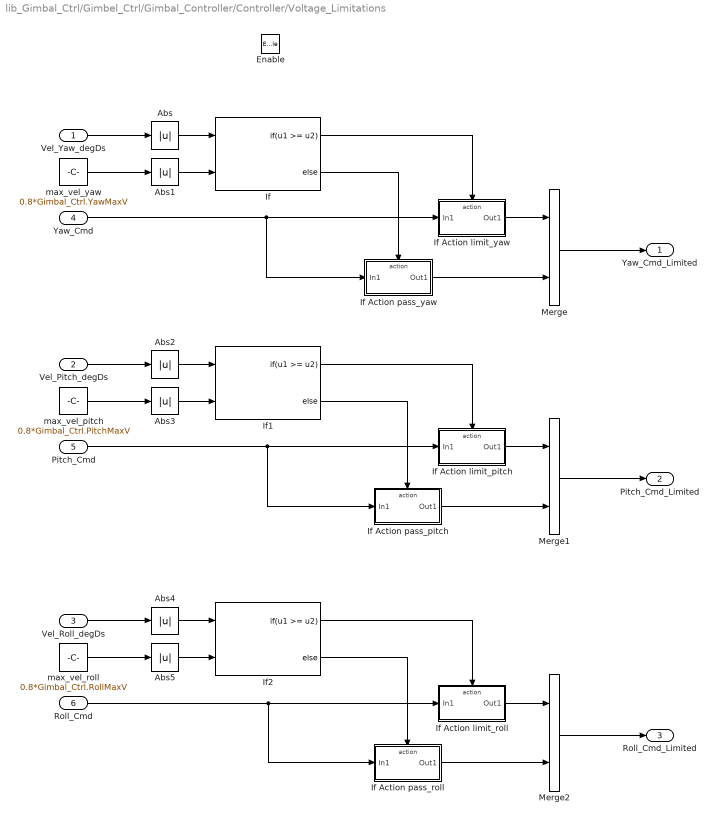
== system lib_Gimbal_Ctrl/Gimbel_Ctrl/Gimbal_Controller/Controller/Voltage_Limitations ==
  Vel_Yaw_degDs : Inport
  Vel_Pitch_degDs : Inport  Port=2
  Vel_Roll_degDs : Inport  Port=3
  Yaw_Cmd : Inport  Port=4
  Pitch_Cmd : Inport  Port=5
  Roll_Cmd : Inport  Port=6
  Enable : EnablePort
  Abs{,1..5} (6 alike) : Abs
  If : If  NumInputs=2  IfExpression=u1 >= u2
  If Action limit_pitch : Subsystem  TreatAsAtomicUnit=on
  If Action limit_roll : Subsystem  TreatAsAtomicUnit=on
  If Action limit_yaw : Subsystem  TreatAsAtomicUnit=on
  If Action pass_pitch : Subsystem  TreatAsAtomicUnit=on
  If Action pass_roll : Subsystem  TreatAsAtomicUnit=on
  If Action pass_yaw : Subsystem  TreatAsAtomicUnit=on
  If1 : If  NumInputs=2  IfExpression=u1 >= u2
  If2 : If  NumInputs=2  IfExpression=u1 >= u2
  Merge : Merge
  Merge1 : Merge
  Merge2 : Merge
  max_vel_pitch : Constant  Value=0.8*Gimbal_Ctrl.PitchMaxV
  max_vel_roll : Constant  Value=0.8*Gimbal_Ctrl.RollMaxV
  max_vel_yaw : Constant  Value=0.8*Gimbal_Ctrl.YawMaxV
  Yaw_Cmd_Limited : Outport
  Pitch_Cmd_Limited : Outport  Port=2
  Roll_Cmd_Limited : Outport  Port=3
  wires:
  max_vel_yaw/1 -> Abs1/1
  Vel_Yaw_degDs/1 -> Abs/1
  Vel_Pitch_degDs/1 -> Abs2/1
  max_vel_pitch/1 -> Abs3/1
  Vel_Roll_degDs/1 -> Abs4/1
  max_vel_roll/1 -> Abs5/1
  If/1 -> If Action limit_yaw/Action
  If/2 -> If Action pass_yaw/Action
  If Action pass_yaw/1(Out1) -> Merge/2
  If Action limit_yaw/1(Out1) -> Merge/1
  Yaw_Cmd/1 -> If Action pass_yaw/1(In1), If Action limit_yaw/1(In1)
  Merge/1 -> Yaw_Cmd_Limited/1
  Pitch_Cmd/1 -> If Action pass_pitch/1(In1), If Action limit_pitch/1(In1)
  If1/1 -> If Action limit_pitch/Action
  If1/2 -> If Action pass_pitch/Action
  If Action limit_pitch/1(Out1) -> Merge1/1
  If Action pass_pitch/1(Out1) -> Merge1/2
  Merge1/1 -> Pitch_Cmd_Limited/1
  Roll_Cmd/1 -> If Action pass_roll/1(In1), If Action limit_roll/1(In1)
  If2/1 -> If Action limit_roll/Action
  If2/2 -> If Action pass_roll/Action
  If Action limit_roll/1(Out1) -> Merge2/1
  If Action pass_roll/1(Out1) -> Merge2/2
  Merge2/1 -> Roll_Cmd_Limited/1
  Abs/1 -> If/1
  Abs1/1 -> If/2
  Abs2/1 -> If1/1
  Abs3/1 -> If1/2
  Abs4/1 -> If2/1
  Abs5/1 -> If2/2

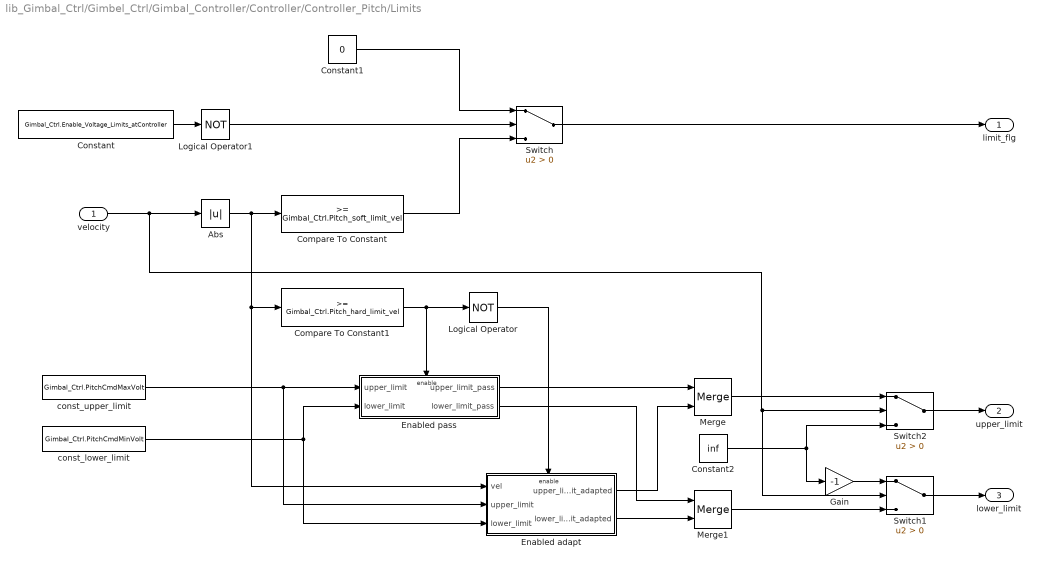
== system lib_Gimbal_Ctrl/Gimbel_Ctrl/Gimbal_Controller/Controller/Controller_Pitch/Limits ==
  velocity : Inport
  Abs : Abs
  Compare To Constant : simulink/Logic and Bit Operations/Compare To Constant  relop=>=  const=Gimbal_Ctrl.Pitch_soft_limit_vel  OutDataTypeStr=boolean
  Compare To Constant1 : simulink/Logic and Bit Operations/Compare To Constant  relop=>=  const=Gimbal_Ctrl.Pitch_hard_limit_vel  OutDataTypeStr=boolean
  Constant : Constant  Value=Gimbal_Ctrl.Enable_Voltage_Limits_atController
  Constant1 : Constant  Value=0  OutDataTypeStr=boolean
  Constant2 : Constant  Value=inf
  Enabled adapt : Subsystem  TreatAsAtomicUnit=on
  Enabled pass : Subsystem  TreatAsAtomicUnit=on
  Gain : Gain  Gain=-1
  Logical Operator : Logic  Operator=NOT  AllPortsSameDT=off  OutDataTypeStr=boolean
  Logical Operator1 : Logic  Operator=NOT  AllPortsSameDT=off  OutDataTypeStr=boolean
  Merge : Merge
  Merge1 : Merge
  Switch : Switch  Criteria=u2 > Threshold
  Switch1 : Switch  Criteria=u2 > Threshold
  Switch2 : Switch  Criteria=u2 > Threshold
  const_lower_limit : Constant  Value=Gimbal_Ctrl.PitchCmdMinVolt
  const_upper_limit : Constant  Value=Gimbal_Ctrl.PitchCmdMaxVolt
  limit_flg : Outport
  upper_limit : Outport  Port=2
  lower_limit : Outport  Port=3
  wires:
  Compare To Constant1/1 -> Logical Operator/1, Enabled pass/Enable
  Abs/1 -> Compare To Constant/1, Compare To Constant1/1, Enabled adapt/1(vel)
  Enabled adapt/1(upper_limit_adapted) -> Merge/2
  Enabled pass/2(lower_limit_pass) -> Merge1/1
  Enabled pass/1(upper_limit_pass) -> Merge/1
  velocity/1 -> Switch1/2, Switch2/2, Abs/1
  Logical Operator/1 -> Enabled adapt/Enable
  const_upper_limit/1 -> Enabled adapt/2(upper_limit), Enabled pass/1(upper_limit)
  const_lower_limit/1 -> Enabled adapt/3(lower_limit), Enabled pass/2(lower_limit)
  Enabled adapt/2(lower_limit_adapted) -> Merge1/2
  Constant1/1 -> Switch/1
  Logical Operator1/1 -> Switch/2
  Constant/1 -> Logical Operator1/1
  Switch/1 -> limit_flg/1
  Compare To Constant/1 -> Switch/3
  Merge/1 -> Switch2/1
  Merge1/1 -> Switch1/3
  Switch1/1 -> lower_limit/1
  Switch2/1 -> upper_limit/1
  Constant2/1 -> Gain/1, Switch2/3
  Gain/1 -> Switch1/1

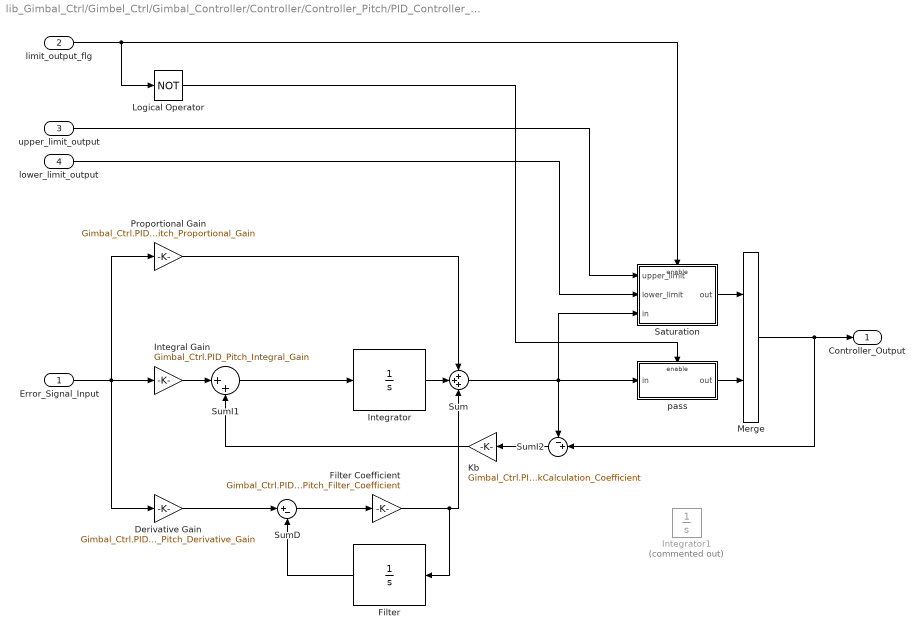
== system lib_Gimbal_Ctrl/Gimbel_Ctrl/Gimbal_Controller/Controller/Controller_Pitch/PID_Controller_Dynamic_Limits ==
  Error_Signal_Input : Inport  SampleTime=SampTime
  limit_output_flg : Inport  Port=2  SampleTime=SampTime
  upper_limit_output : Inport  Port=3  SampleTime=SampTime
  lower_limit_output : Inport  Port=4  SampleTime=SampTime
  Derivative Gain : Gain  DisableCoverage=on  Gain=Gimbal_Ctrl.PID_Pitch_Derivative_Gain  SampleTime=Gimbal_Ctrl.SampTime
  Filter : Integrator  DisableCoverage=on
  Filter Coefficient : Gain  Gain=Gimbal_Ctrl.PID_Pitch_Filter_Coefficient  SampleTime=Gimbal_Ctrl.SampTime
  Integral Gain : Gain  DisableCoverage=on  Gain=Gimbal_Ctrl.PID_Pitch_Integral_Gain  SampleTime=Gimbal_Ctrl.SampTime
  Integrator : Integrator
  Integrator1 : Integrator  Commented=on
  Kb : Gain  Gain=Gimbal_Ctrl.PID_Pitch_BackCalculation_Coefficient  SaturateOnIntegerOverflow=on
  Logical Operator : Logic  Operator=NOT  AllPortsSameDT=off  OutDataTypeStr=boolean
  Merge : Merge
  Proportional Gain : Gain  Gain=Gimbal_Ctrl.PID_Pitch_Proportional_Gain  SampleTime=Gimbal_Ctrl.SampTime
  Saturation : Subsystem
  Sum : Sum  Inputs=+++  SampleTime=SampTime
  SumD : Sum  DisableCoverage=on  Inputs=|+-  SampleTime=SampTime
  SumI1 : Sum  Inputs=|++  SaturateOnIntegerOverflow=on
  SumI2 : Sum  DisableCoverage=on  Inputs=-+|  SaturateOnIntegerOverflow=on
  pass : Subsystem
  Controller_Output : Outport  SampleTime=SampTime  InitialOutput=0
  wires:
  Kb/1 -> SumI1/2
  Merge/1 -> Controller_Output/1, SumI2/2
  Derivative Gain/1 -> SumD/1
  Filter/1 -> SumD/2
  SumD/1 -> Filter Coefficient/1
  Integrator/1 -> Sum/2
  Filter Coefficient/1 -> Filter/1, Sum/3
  SumI1/1 -> Integrator/1
  SumI2/1 -> Kb/1
  Sum/1 -> Saturation/3(in), pass/1(in), SumI2/1
  Proportional Gain/1 -> Sum/1
  Error_Signal_Input/1 -> Integral Gain/1, Derivative Gain/1, Proportional Gain/1
  Integral Gain/1 -> SumI1/1
  Saturation/1(out) -> Merge/1
  pass/1(out) -> Merge/2
  lower_limit_output/1 -> Saturation/2(lower_limit)
  upper_limit_output/1 -> Saturation/1(upper_limit)
  limit_output_flg/1 -> Logical Operator/1, Saturation/Enable
  Logical Operator/1 -> pass/Enable

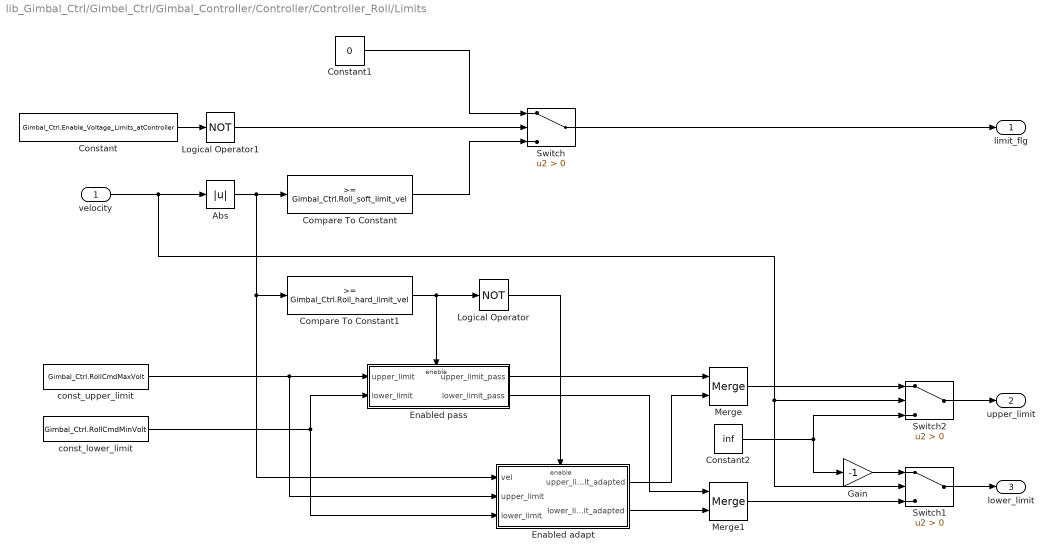
== system lib_Gimbal_Ctrl/Gimbel_Ctrl/Gimbal_Controller/Controller/Controller_Roll/Limits ==
  velocity : Inport
  Abs : Abs
  Compare To Constant : simulink/Logic and Bit Operations/Compare To Constant  relop=>=  const=Gimbal_Ctrl.Roll_soft_limit_vel  OutDataTypeStr=boolean
  Compare To Constant1 : simulink/Logic and Bit Operations/Compare To Constant  relop=>=  const=Gimbal_Ctrl.Roll_hard_limit_vel  OutDataTypeStr=boolean
  Constant : Constant  Value=Gimbal_Ctrl.Enable_Voltage_Limits_atController
  Constant1 : Constant  Value=0  OutDataTypeStr=boolean
  Constant2 : Constant  Value=inf
  Enabled adapt : Subsystem  TreatAsAtomicUnit=on
  Enabled pass : Subsystem  TreatAsAtomicUnit=on
  Gain : Gain  Gain=-1
  Logical Operator : Logic  Operator=NOT  AllPortsSameDT=off  OutDataTypeStr=boolean
  Logical Operator1 : Logic  Operator=NOT  AllPortsSameDT=off  OutDataTypeStr=boolean
  Merge : Merge
  Merge1 : Merge
  Switch : Switch  Criteria=u2 > Threshold
  Switch1 : Switch  Criteria=u2 > Threshold
  Switch2 : Switch  Criteria=u2 > Threshold
  const_lower_limit : Constant  Value=Gimbal_Ctrl.RollCmdMinVolt
  const_upper_limit : Constant  Value=Gimbal_Ctrl.RollCmdMaxVolt
  limit_flg : Outport
  upper_limit : Outport  Port=2
  lower_limit : Outport  Port=3
  wires:
  Compare To Constant1/1 -> Logical Operator/1, Enabled pass/Enable
  Abs/1 -> Compare To Constant/1, Compare To Constant1/1, Enabled adapt/1(vel)
  Enabled adapt/1(upper_limit_adapted) -> Merge/2
  Enabled pass/2(lower_limit_pass) -> Merge1/1
  Enabled pass/1(upper_limit_pass) -> Merge/1
  velocity/1 -> Switch2/2, Switch1/2, Abs/1
  Logical Operator/1 -> Enabled adapt/Enable
  const_upper_limit/1 -> Enabled adapt/2(upper_limit), Enabled pass/1(upper_limit)
  const_lower_limit/1 -> Enabled adapt/3(lower_limit), Enabled pass/2(lower_limit)
  Enabled adapt/2(lower_limit_adapted) -> Merge1/2
  Constant1/1 -> Switch/1
  Logical Operator1/1 -> Switch/2
  Constant/1 -> Logical Operator1/1
  Switch/1 -> limit_flg/1
  Compare To Constant/1 -> Switch/3
  Merge/1 -> Switch2/1
  Merge1/1 -> Switch1/3
  Gain/1 -> Switch1/1
  Constant2/1 -> Gain/1, Switch2/3
  Switch2/1 -> upper_limit/1
  Switch1/1 -> lower_limit/1

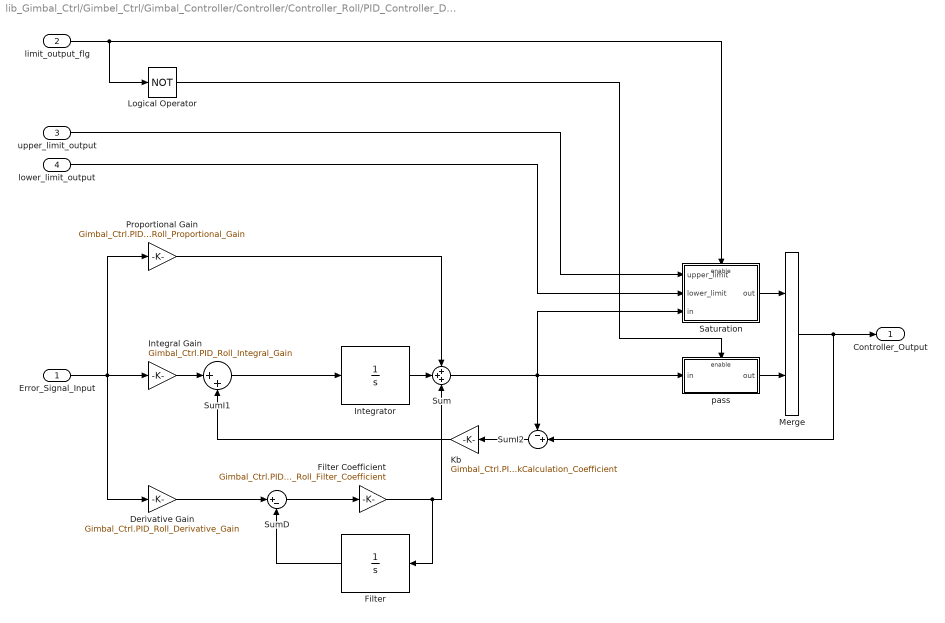
== system lib_Gimbal_Ctrl/Gimbel_Ctrl/Gimbal_Controller/Controller/Controller_Roll/PID_Controller_Dynamic_Limits ==
  Error_Signal_Input : Inport  SampleTime=SampTime
  limit_output_flg : Inport  Port=2  SampleTime=SampTime
  upper_limit_output : Inport  Port=3  SampleTime=SampTime
  lower_limit_output : Inport  Port=4  SampleTime=SampTime
  Derivative Gain : Gain  DisableCoverage=on  Gain=Gimbal_Ctrl.PID_Roll_Derivative_Gain  SampleTime=Gimbal_Ctrl.SampTime
  Filter : Integrator  DisableCoverage=on
  Filter Coefficient : Gain  Gain=Gimbal_Ctrl.PID_Roll_Filter_Coefficient  SampleTime=Gimbal_Ctrl.SampTime
  Integral Gain : Gain  DisableCoverage=on  Gain=Gimbal_Ctrl.PID_Roll_Integral_Gain  SampleTime=Gimbal_Ctrl.SampTime
  Integrator : Integrator
  Kb : Gain  Gain=Gimbal_Ctrl.PID_Roll_BackCalculation_Coefficient  SaturateOnIntegerOverflow=on
  Logical Operator : Logic  Operator=NOT  AllPortsSameDT=off  OutDataTypeStr=boolean
  Merge : Merge
  Proportional Gain : Gain  Gain=Gimbal_Ctrl.PID_Roll_Proportional_Gain  SampleTime=Gimbal_Ctrl.SampTime
  Saturation : Subsystem
  Sum : Sum  Inputs=+++  SampleTime=SampTime
  SumD : Sum  DisableCoverage=on  Inputs=|+-  SampleTime=SampTime
  SumI1 : Sum  Inputs=|++  SaturateOnIntegerOverflow=on
  SumI2 : Sum  DisableCoverage=on  Inputs=-+|  SaturateOnIntegerOverflow=on
  pass : Subsystem
  Controller_Output : Outport  SampleTime=SampTime  InitialOutput=0
  wires:
  Kb/1 -> SumI1/2
  Merge/1 -> Controller_Output/1, SumI2/2
  Derivative Gain/1 -> SumD/1
  Filter/1 -> SumD/2
  SumD/1 -> Filter Coefficient/1
  Integrator/1 -> Sum/2
  Filter Coefficient/1 -> Filter/1, Sum/3
  SumI1/1 -> Integrator/1
  SumI2/1 -> Kb/1
  Sum/1 -> Saturation/3(in), pass/1(in), SumI2/1
  Proportional Gain/1 -> Sum/1
  Error_Signal_Input/1 -> Integral Gain/1, Derivative Gain/1, Proportional Gain/1
  Integral Gain/1 -> SumI1/1
  Saturation/1(out) -> Merge/1
  pass/1(out) -> Merge/2
  upper_limit_output/1 -> Saturation/1(upper_limit)
  lower_limit_output/1 -> Saturation/2(lower_limit)
  limit_output_flg/1 -> Saturation/Enable, Logical Operator/1
  Logical Operator/1 -> pass/Enable

== system lib_Gimbal_Ctrl/Gimbel_Ctrl/Gimbal_Controller/Controller/Controller_Yaw/Limit_Controllers ==
  Controller_Cmd : Inport
  Velocity : Inport  Port=2
  Constant : Constant  Value=Gimbal_Ctrl.Enable_Limit_Controllers
  Control_Limits : Subsystem
  Logical Operator : Logic  Operator=NOT  AllPortsSameDT=off  OutDataTypeStr=boolean
  Merge : Merge
  pass : Subsystem
  Output : Outport
  wires:
  Controller_Cmd/1 -> Control_Limits/1(Controller_Cmd), pass/1(Controller_Cmd)
  Constant/1 -> Control_Limits/Enable, Logical Operator/1
  Logical Operator/1 -> pass/Enable
  Velocity/1 -> Control_Limits/2(Velocity)
  Control_Limits/1(Output) -> Merge/2
  pass/1(Output) -> Merge/1
  Merge/1 -> Output/1

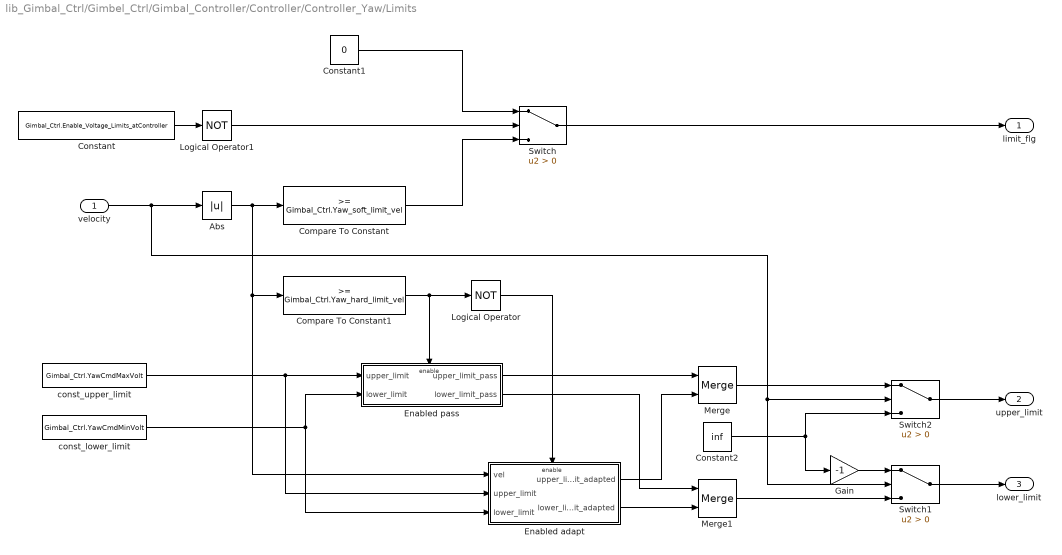
== system lib_Gimbal_Ctrl/Gimbel_Ctrl/Gimbal_Controller/Controller/Controller_Yaw/Limits ==
  velocity : Inport
  Abs : Abs
  Compare To Constant : simulink/Logic and Bit Operations/Compare To Constant  relop=>=  const=Gimbal_Ctrl.Yaw_soft_limit_vel  OutDataTypeStr=boolean
  Compare To Constant1 : simulink/Logic and Bit Operations/Compare To Constant  relop=>=  const=Gimbal_Ctrl.Yaw_hard_limit_vel  OutDataTypeStr=boolean
  Constant : Constant  Value=Gimbal_Ctrl.Enable_Voltage_Limits_atController
  Constant1 : Constant  Value=0  OutDataTypeStr=boolean
  Constant2 : Constant  Value=inf
  Enabled adapt : Subsystem  TreatAsAtomicUnit=on
  Enabled pass : Subsystem  TreatAsAtomicUnit=on
  Gain : Gain  Gain=-1
  Logical Operator : Logic  Operator=NOT  AllPortsSameDT=off  OutDataTypeStr=boolean
  Logical Operator1 : Logic  Operator=NOT  AllPortsSameDT=off  OutDataTypeStr=boolean
  Merge : Merge
  Merge1 : Merge
  Switch : Switch  Criteria=u2 > Threshold
  Switch1 : Switch  Criteria=u2 > Threshold
  Switch2 : Switch  Criteria=u2 > Threshold
  const_lower_limit : Constant  Value=Gimbal_Ctrl.YawCmdMinVolt
  const_upper_limit : Constant  Value=Gimbal_Ctrl.YawCmdMaxVolt
  limit_flg : Outport
  upper_limit : Outport  Port=2
  lower_limit : Outport  Port=3
  wires:
  Compare To Constant1/1 -> Logical Operator/1, Enabled pass/Enable
  Abs/1 -> Compare To Constant/1, Compare To Constant1/1, Enabled adapt/1(vel)
  Enabled adapt/1(upper_limit_adapted) -> Merge/2
  Enabled pass/2(lower_limit_pass) -> Merge1/1
  Enabled pass/1(upper_limit_pass) -> Merge/1
  velocity/1 -> Switch1/2, Switch2/2, Abs/1
  Logical Operator/1 -> Enabled adapt/Enable
  const_upper_limit/1 -> Enabled adapt/2(upper_limit), Enabled pass/1(upper_limit)
  const_lower_limit/1 -> Enabled adapt/3(lower_limit), Enabled pass/2(lower_limit)
  Enabled adapt/2(lower_limit_adapted) -> Merge1/2
  Constant/1 -> Logical Operator1/1
  Logical Operator1/1 -> Switch/2
  Switch/1 -> limit_flg/1
  Compare To Constant/1 -> Switch/3
  Constant1/1 -> Switch/1
  Merge/1 -> Switch2/1
  Merge1/1 -> Switch1/3
  Constant2/1 -> Switch2/3, Gain/1
  Switch1/1 -> lower_limit/1
  Switch2/1 -> upper_limit/1
  Gain/1 -> Switch1/1

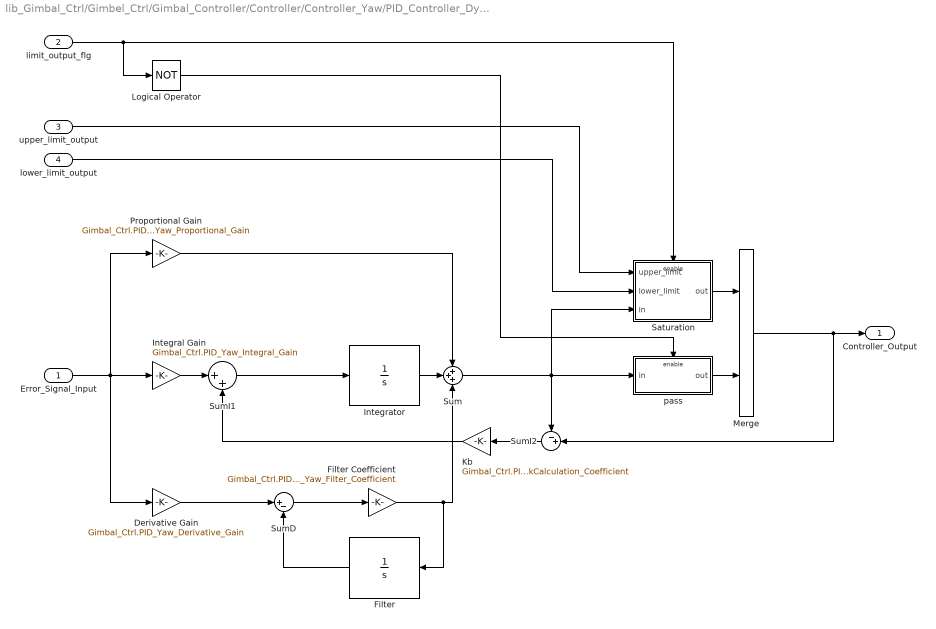
== system lib_Gimbal_Ctrl/Gimbel_Ctrl/Gimbal_Controller/Controller/Controller_Yaw/PID_Controller_Dynamic_Limits ==
  Error_Signal_Input : Inport  SampleTime=Gimbal_Ctrl.SampTime
  limit_output_flg : Inport  Port=2  SampleTime=SampTime
  upper_limit_output : Inport  Port=3  SampleTime=SampTime
  lower_limit_output : Inport  Port=4  SampleTime=SampTime
  Derivative Gain : Gain  DisableCoverage=on  Gain=Gimbal_Ctrl.PID_Yaw_Derivative_Gain  SampleTime=Gimbal_Ctrl.SampTime
  Filter : Integrator  DisableCoverage=on
  Filter Coefficient : Gain  Gain=Gimbal_Ctrl.PID_Yaw_Filter_Coefficient  SampleTime=Gimbal_Ctrl.SampTime
  Integral Gain : Gain  DisableCoverage=on  Gain=Gimbal_Ctrl.PID_Yaw_Integral_Gain  SampleTime=Gimbal_Ctrl.SampTime
  Integrator : Integrator
  Kb : Gain  Gain=Gimbal_Ctrl.PID_Yaw_BackCalculation_Coefficient  SaturateOnIntegerOverflow=on
  Logical Operator : Logic  Operator=NOT  AllPortsSameDT=off  OutDataTypeStr=boolean
  Merge : Merge
  Proportional Gain : Gain  Gain=Gimbal_Ctrl.PID_Yaw_Proportional_Gain  SampleTime=Gimbal_Ctrl.SampTime
  Saturation : Subsystem
  Sum : Sum  Inputs=+++  SampleTime=SampTime
  SumD : Sum  DisableCoverage=on  Inputs=|+-  SampleTime=SampTime
  SumI1 : Sum  Inputs=|++  SaturateOnIntegerOverflow=on
  SumI2 : Sum  DisableCoverage=on  Inputs=-+|  SaturateOnIntegerOverflow=on
  pass : Subsystem
  Controller_Output : Outport  SampleTime=SampTime  InitialOutput=0
  wires:
  Kb/1 -> SumI1/2
  Derivative Gain/1 -> SumD/1
  Filter/1 -> SumD/2
  SumD/1 -> Filter Coefficient/1
  Integrator/1 -> Sum/2
  Filter Coefficient/1 -> Filter/1, Sum/3
  SumI1/1 -> Integrator/1
  SumI2/1 -> Kb/1
  Sum/1 -> pass/1(in), Saturation/3(in), SumI2/1
  Proportional Gain/1 -> Sum/1
  Error_Signal_Input/1 -> Integral Gain/1, Derivative Gain/1, Proportional Gain/1
  Integral Gain/1 -> SumI1/1
  Merge/1 -> Controller_Output/1, SumI2/2
  pass/1(out) -> Merge/2
  Saturation/1(out) -> Merge/1
  upper_limit_output/1 -> Saturation/1(upper_limit)
  lower_limit_output/1 -> Saturation/2(lower_limit)
  limit_output_flg/1 -> Logical Operator/1, Saturation/Enable
  Logical Operator/1 -> pass/Enable

== system lib_Gimbal_Ctrl/Gimbel_Ctrl/Gimbal_Controller/Controller/Monitor_Velocity_Limits/Pitch_rate_limit ==
  note: need to chack the critical value of u1
  "Input " : Inport
  Abs : Abs
  Constant : Constant
  Constant1 : Constant  Value=Gimbal_Ctrl.PitchMaxV
  Gain : Gain  Gain=1/Gimbal_Ctrl.MaxCheck
  If : If  NumInputs=2  IfExpression=u1 >u2
  If Action Subsystem : Subsystem  TreatAsAtomicUnit=on
  If Action Subsystem1 : Subsystem  TreatAsAtomicUnit=on
  Sum : Sum  Inputs=|+-
  Transport Delay : TransportDelay  DelayTime=Gimbal_Ctrl.MaxCheck
  Velocity_pitch : Scope
  Pitch_vel_degDs : Outport
  StopSim : Outport  Port=2
  Continue : Outport  Port=3
  wires:
  "Input "/1 -> If Action Subsystem/1(In1), Transport Delay/1, Sum/1
  Transport Delay/1 -> Sum/2
  Sum/1 -> Gain/1
  If/2 -> If Action Subsystem/Action
  If/1 -> If Action Subsystem1/Action
  If Action Subsystem1/1(Out1) -> StopSim/1
  If Action Subsystem/1(Out1) -> Continue/1
  Constant/1 -> If Action Subsystem1/1(In1)
  Gain/1 -> Velocity_pitch/1, Pitch_vel_degDs/1, Abs/1
  Constant1/1 -> If/2
  Abs/1 -> If/1

== system lib_Gimbal_Ctrl/Gimbel_Ctrl/Gimbal_Controller/Controller/Monitor_Velocity_Limits/Roll_Rate_limit ==
  note: need to chack the critical value of u1
  "Input " : Inport
  Abs : Abs
  Constant : Constant
  Constant1 : Constant  Value=Gimbal_Ctrl.RollMaxV
  Gain : Gain  Gain=1/Gimbal_Ctrl.MaxCheck
  If : If  NumInputs=2  IfExpression=u1 >u2
  If Action Subsystem : Subsystem  TreatAsAtomicUnit=on
  If Action Subsystem1 : Subsystem  TreatAsAtomicUnit=on
  Sum : Sum  Inputs=|+-
  Transport Delay : TransportDelay  DelayTime=Gimbal_Ctrl.MaxCheck
  Velocity_roll : Scope
  Roll_vel_degDs : Outport
  StopSim : Outport  Port=2
  Continue : Outport  Port=3
  wires:
  "Input "/1 -> If Action Subsystem/1(In1), Transport Delay/1, Sum/1
  Transport Delay/1 -> Sum/2
  Sum/1 -> Gain/1
  If/2 -> If Action Subsystem/Action
  If/1 -> If Action Subsystem1/Action
  If Action Subsystem1/1(Out1) -> StopSim/1
  If Action Subsystem/1(Out1) -> Continue/1
  Constant/1 -> If Action Subsystem1/1(In1)
  Gain/1 -> Roll_vel_degDs/1, Velocity_roll/1, Abs/1
  Constant1/1 -> If/2
  Abs/1 -> If/1

== system lib_Gimbal_Ctrl/Gimbel_Ctrl/Gimbal_Controller/Controller/Monitor_Velocity_Limits/Yaw_rate_limit ==
  note: need to check the critical value of u1
  "Input " : Inport
  Abs : Abs
  Constant : Constant
  Constant1 : Constant  Value=Gimbal_Ctrl.YawMaxV
  Gain : Gain  Gain=1/Gimbal_Ctrl.MaxCheck
  If : If  NumInputs=2  IfExpression=u1 > u2
  If Action Subsystem : Subsystem  TreatAsAtomicUnit=on
  If Action Subsystem1 : Subsystem  TreatAsAtomicUnit=on
  Sum : Sum  Inputs=|+-
  Transport Delay : TransportDelay  DelayTime=Gimbal_Ctrl.MaxCheck
  velocity_yaw : Scope
  Yaw_vel_degDs : Outport
  StopSim : Outport  Port=2
  Continue : Outport  Port=3
  wires:
  "Input "/1 -> If Action Subsystem/1(In1), Transport Delay/1, Sum/1
  Transport Delay/1 -> Sum/2
  Sum/1 -> Gain/1
  If/2 -> If Action Subsystem/Action
  If/1 -> If Action Subsystem1/Action
  If Action Subsystem1/1(Out1) -> StopSim/1
  If Action Subsystem/1(Out1) -> Continue/1
  Constant/1 -> If Action Subsystem1/1(In1)
  Gain/1 -> Yaw_vel_degDs/1, velocity_yaw/1, Abs/1
  Constant1/1 -> If/2
  Abs/1 -> If/1

== system lib_Gimbal_Ctrl/Gimbel_Ctrl/Gimbal_Controller/Controller/Voltage_Limitations/If Action limit_pitch ==
  In1 : Inport
  Action Port : ActionPort
  Limit_Voltage_Pitch : Saturate  UpperLimit=Gimbal_Ctrl.PitchCmdMaxVolt  LowerLimit=-Gimbal_Ctrl.PitchCmdMaxVolt
  Out1 : Outport
  wires:
  In1/1 -> Limit_Voltage_Pitch/1
  Limit_Voltage_Pitch/1 -> Out1/1

== system lib_Gimbal_Ctrl/Gimbel_Ctrl/Gimbal_Controller/Controller/Voltage_Limitations/If Action limit_roll ==
  In1 : Inport
  Action Port : ActionPort
  Limit_Voltage_Roll : Saturate  UpperLimit=Gimbal_Ctrl.RollCmdMaxVolt  LowerLimit=-Gimbal_Ctrl.RollCmdMaxVolt
  Out1 : Outport
  wires:
  In1/1 -> Limit_Voltage_Roll/1
  Limit_Voltage_Roll/1 -> Out1/1

== system lib_Gimbal_Ctrl/Gimbel_Ctrl/Gimbal_Controller/Controller/Voltage_Limitations/If Action limit_yaw ==
  In1 : Inport
  Action Port : ActionPort
  Limit_Voltage_Yaw : Saturate  UpperLimit=Gimbal_Ctrl.YawCmdMaxVolt  LowerLimit=-Gimbal_Ctrl.YawCmdMaxVolt
  Out1 : Outport
  wires:
  In1/1 -> Limit_Voltage_Yaw/1
  Limit_Voltage_Yaw/1 -> Out1/1

== system lib_Gimbal_Ctrl/Gimbel_Ctrl/Gimbal_Controller/Controller/Voltage_Limitations/If Action pass_pitch ==
  In1 : Inport
  Action Port : ActionPort
  Out1 : Outport
  wires:
  In1/1 -> Out1/1

== system lib_Gimbal_Ctrl/Gimbel_Ctrl/Gimbal_Controller/Controller/Voltage_Limitations/If Action pass_roll ==
  In1 : Inport
  Action Port : ActionPort
  Out1 : Outport
  wires:
  In1/1 -> Out1/1

== system lib_Gimbal_Ctrl/Gimbel_Ctrl/Gimbal_Controller/Controller/Voltage_Limitations/If Action pass_yaw ==
  In1 : Inport
  Action Port : ActionPort
  Out1 : Outport
  wires:
  In1/1 -> Out1/1

== system lib_Gimbal_Ctrl/Gimbel_Ctrl/Gimbal_Controller/Controller/Controller_Pitch/Limits/Enabled adapt ==
  vel : Inport
  upper_limit : Inport  Port=2
  lower_limit : Inport  Port=3
  Enable : EnablePort
  Abs : Abs
  Add : Sum  Inputs=+-
  Constant : Constant  Value=Gimbal_Ctrl.Pitch_hard_limit_vel
  Constant1 : Constant  Value=Gimbal_Ctrl.Pitch_limit_adaption_coef-1
  Divide : Product  Inputs=*/
  Gain : Gain  Gain=Gimbal_Ctrl.Pitch_limit_adaption_coef
  Product : Product
  Product1 : Product
  upper_limit_adapted : Outport
  lower_limit_adapted : Outport  Port=2
  wires:
  Constant/1 -> Abs/1
  Abs/1 -> Divide/1
  vel/1 -> Divide/2
  Divide/1 -> Gain/1
  Gain/1 -> Add/1
  Constant1/1 -> Add/2
  upper_limit/1 -> Product/2
  Add/1 -> Product/1, Product1/1
  Product/1 -> upper_limit_adapted/1
  lower_limit/1 -> Product1/2
  Product1/1 -> lower_limit_adapted/1
